simulink model "Filter_Fixed"  (R2017b)
settings: Solver=FixedStepDiscrete  StartTime=0.0  StopTime=400  RelTol=1e-3
undefined symbols (not defined in the file or in its folder): designMultirateFIR
libraries: dspmlti4 x1
(part 3 of 3)

== system Filter_Fixed/HighpassH/Resonator75 ==
  In1 : Inport
  Delay : Delay  DelayLength=1
  Gain : Gain  Gain=-0.9536+0.30107i  OutDataTypeStr=fixdt(1,24,23)
  GainH : Gain  Gain=-0.16604-0.98612i  OutDataTypeStr=fixdt(1,24,23)
  Sum1 : Sum  Inputs=|++
  Out1 : Outport
  wires:
  In1/1 -> Sum1/1
  GainH/1 -> Out1/1
  Gain/1 -> Sum1/2
  Delay/1 -> Gain/1
  Sum1/1 -> Delay/1, GainH/1

== system Filter_Fixed/HighpassH/Resonator76 ==
  In1 : Inport
  Delay : Delay  DelayLength=1
  Gain : Gain  Gain=-0.9616+0.27445i  OutDataTypeStr=fixdt(1,24,23)
  GainH : Gain  Gain=0.15231+0.98833i  OutDataTypeStr=fixdt(1,24,23)
  Sum1 : Sum  Inputs=|++
  Out1 : Outport
  wires:
  In1/1 -> Sum1/1
  GainH/1 -> Out1/1
  Gain/1 -> Sum1/2
  Delay/1 -> Gain/1
  Sum1/1 -> Delay/1, GainH/1

== system Filter_Fixed/HighpassH/Resonator77 ==
  In1 : Inport
  Delay : Delay  DelayLength=1
  Gain : Gain  Gain=-0.96886+0.24761i  OutDataTypeStr=fixdt(1,24,23)
  GainH : Gain  Gain=-0.13856-0.99035i  OutDataTypeStr=fixdt(1,24,23)
  Sum1 : Sum  Inputs=|++
  Out1 : Outport
  wires:
  In1/1 -> Sum1/1
  GainH/1 -> Out1/1
  Gain/1 -> Sum1/2
  Delay/1 -> Gain/1
  Sum1/1 -> Delay/1, GainH/1

== system Filter_Fixed/HighpassH/Resonator78 ==
  In1 : Inport
  Delay : Delay  DelayLength=1
  Gain : Gain  Gain=-0.97537+0.22058i  OutDataTypeStr=fixdt(1,24,23)
  GainH : Gain  Gain=0.12478+0.99218i  OutDataTypeStr=fixdt(1,24,23)
  Sum1 : Sum  Inputs=|++
  Out1 : Outport
  wires:
  In1/1 -> Sum1/1
  GainH/1 -> Out1/1
  Gain/1 -> Sum1/2
  Delay/1 -> Gain/1
  Sum1/1 -> Delay/1, GainH/1

== system Filter_Fixed/HighpassH/Resonator79 ==
  In1 : Inport
  Delay : Delay  DelayLength=1
  Gain : Gain  Gain=-0.98112+0.19339i  OutDataTypeStr=fixdt(1,24,23)
  GainH : Gain  Gain=-0.11098-0.99382i  OutDataTypeStr=fixdt(1,24,23)
  Sum1 : Sum  Inputs=|++
  Out1 : Outport
  wires:
  In1/1 -> Sum1/1
  GainH/1 -> Out1/1
  Gain/1 -> Sum1/2
  Delay/1 -> Gain/1
  Sum1/1 -> Delay/1, GainH/1

== system Filter_Fixed/HighpassH/Resonator8 ==
  In1 : Inport
  Delay : Delay  DelayLength=1
  Gain : Gain  Gain=0.56277+0.82661i  OutDataTypeStr=fixdt(1,24,23)
  GainH : Gain  Gain=0.89037+0.45523i  OutDataTypeStr=fixdt(1,24,23)
  Sum1 : Sum  Inputs=|++
  Out1 : Outport
  wires:
  In1/1 -> Sum1/1
  GainH/1 -> Out1/1
  Gain/1 -> Sum1/2
  Delay/1 -> Gain/1
  Sum1/1 -> Delay/1, GainH/1

== system Filter_Fixed/HighpassH/Resonator80 ==
  In1 : Inport
  Delay : Delay  DelayLength=1
  Gain : Gain  Gain=-0.98612+0.16604i  OutDataTypeStr=fixdt(1,24,23)
  GainH : Gain  Gain=0.097152+0.99527i  OutDataTypeStr=fixdt(1,24,23)
  Sum1 : Sum  Inputs=|++
  Out1 : Outport
  wires:
  In1/1 -> Sum1/1
  GainH/1 -> Out1/1
  Gain/1 -> Sum1/2
  Delay/1 -> Gain/1
  Sum1/1 -> Delay/1, GainH/1

== system Filter_Fixed/HighpassH/Resonator81 ==
  In1 : Inport
  Delay : Delay  DelayLength=1
  Gain : Gain  Gain=-0.99035+0.13856i  OutDataTypeStr=fixdt(1,24,23)
  GainH : Gain  Gain=-0.083308-0.99652i  OutDataTypeStr=fixdt(1,24,23)
  Sum1 : Sum  Inputs=|++
  Out1 : Outport
  wires:
  In1/1 -> Sum1/1
  GainH/1 -> Out1/1
  Gain/1 -> Sum1/2
  Delay/1 -> Gain/1
  Sum1/1 -> Delay/1, GainH/1

== system Filter_Fixed/HighpassH/Resonator82 ==
  In1 : Inport
  Delay : Delay  DelayLength=1
  Gain : Gain  Gain=-0.99382+0.11098i  OutDataTypeStr=fixdt(1,24,23)
  GainH : Gain  Gain=0.069448+0.99759i  OutDataTypeStr=fixdt(1,24,23)
  Sum1 : Sum  Inputs=|++
  Out1 : Outport
  wires:
  In1/1 -> Sum1/1
  GainH/1 -> Out1/1
  Gain/1 -> Sum1/2
  Delay/1 -> Gain/1
  Sum1/1 -> Delay/1, GainH/1

== system Filter_Fixed/HighpassH/Resonator83 ==
  In1 : Inport
  Delay : Delay  DelayLength=1
  Gain : Gain  Gain=-0.99652+0.083308i  OutDataTypeStr=fixdt(1,24,23)
  GainH : Gain  Gain=-0.055575-0.99845i  OutDataTypeStr=fixdt(1,24,23)
  Sum1 : Sum  Inputs=|++
  Out1 : Outport
  wires:
  In1/1 -> Sum1/1
  GainH/1 -> Out1/1
  Gain/1 -> Sum1/2
  Delay/1 -> Gain/1
  Sum1/1 -> Delay/1, GainH/1

== system Filter_Fixed/HighpassH/Resonator84 ==
  In1 : Inport
  Delay : Delay  DelayLength=1
  Gain : Gain  Gain=-0.99845+0.055575i  OutDataTypeStr=fixdt(1,24,23)
  GainH : Gain  Gain=0.04169+0.99913i  OutDataTypeStr=fixdt(1,24,23)
  Sum1 : Sum  Inputs=|++
  Out1 : Outport
  wires:
  In1/1 -> Sum1/1
  GainH/1 -> Out1/1
  Gain/1 -> Sum1/2
  Delay/1 -> Gain/1
  Sum1/1 -> Delay/1, GainH/1

== system Filter_Fixed/HighpassH/Resonator85 ==
  In1 : Inport
  Delay : Delay  DelayLength=1
  Gain : Gain  Gain=-0.99961+0.027798i  OutDataTypeStr=fixdt(1,24,23)
  GainH : Gain  Gain=-0.027798-0.99961i  OutDataTypeStr=fixdt(1,24,23)
  Sum1 : Sum  Inputs=|++
  Out1 : Outport
  wires:
  In1/1 -> Sum1/1
  GainH/1 -> Out1/1
  Gain/1 -> Sum1/2
  Delay/1 -> Gain/1
  Sum1/1 -> Delay/1, GainH/1

== system Filter_Fixed/HighpassH/Resonator86 ==
  In1 : Inport
  Delay : Delay  DelayLength=1
  Gain : Gain  Gain=-1+1.2246e-16i  OutDataTypeStr=fixdt(1,24,23)
  GainH : Gain  Gain=0.0139+0.9999i  OutDataTypeStr=fixdt(1,24,23)
  Sum1 : Sum  Inputs=|++
  Out1 : Outport
  wires:
  In1/1 -> Sum1/1
  GainH/1 -> Out1/1
  Gain/1 -> Sum1/2
  Delay/1 -> Gain/1
  Sum1/1 -> Delay/1, GainH/1

== system Filter_Fixed/HighpassH/Resonator87 ==
  In1 : Inport
  Delay : Delay  DelayLength=1
  Gain : Gain  Gain=-0.99961-0.027798i  OutDataTypeStr=fixdt(1,24,23)
  GainH : Gain  Gain=1.9106e-14-1i  OutDataTypeStr=fixdt(1,24,23)
  Sum1 : Sum  Inputs=|++
  Out1 : Outport
  wires:
  In1/1 -> Sum1/1
  GainH/1 -> Out1/1
  Gain/1 -> Sum1/2
  Delay/1 -> Gain/1
  Sum1/1 -> Delay/1, GainH/1

== system Filter_Fixed/HighpassH/Resonator88 ==
  In1 : Inport
  Delay : Delay  DelayLength=1
  Gain : Gain  Gain=-0.99845-0.055575i  OutDataTypeStr=fixdt(1,24,23)
  GainH : Gain  Gain=0.0139-0.9999i  OutDataTypeStr=fixdt(1,24,23)
  Sum1 : Sum  Inputs=|++
  Out1 : Outport
  wires:
  In1/1 -> Sum1/1
  GainH/1 -> Out1/1
  Gain/1 -> Sum1/2
  Delay/1 -> Gain/1
  Sum1/1 -> Delay/1, GainH/1

== system Filter_Fixed/HighpassH/Resonator89 ==
  In1 : Inport
  Delay : Delay  DelayLength=1
  Gain : Gain  Gain=-0.99652-0.083308i  OutDataTypeStr=fixdt(1,24,23)
  GainH : Gain  Gain=-0.027798+0.99961i  OutDataTypeStr=fixdt(1,24,23)
  Sum1 : Sum  Inputs=|++
  Out1 : Outport
  wires:
  In1/1 -> Sum1/1
  GainH/1 -> Out1/1
  Gain/1 -> Sum1/2
  Delay/1 -> Gain/1
  Sum1/1 -> Delay/1, GainH/1

== system Filter_Fixed/HighpassH/Resonator9 ==
  In1 : Inport
  Delay : Delay  DelayLength=1
  Gain : Gain  Gain=0.53958+0.84194i  OutDataTypeStr=fixdt(1,24,23)
  GainH : Gain  Gain=-0.88396-0.46756i  OutDataTypeStr=fixdt(1,24,23)
  Sum1 : Sum  Inputs=|++
  Out1 : Outport
  wires:
  In1/1 -> Sum1/1
  GainH/1 -> Out1/1
  Gain/1 -> Sum1/2
  Delay/1 -> Gain/1
  Sum1/1 -> Delay/1, GainH/1

== system Filter_Fixed/HighpassH/Resonator90 ==
  In1 : Inport
  Delay : Delay  DelayLength=1
  Gain : Gain  Gain=-0.99382-0.11098i  OutDataTypeStr=fixdt(1,24,23)
  GainH : Gain  Gain=0.04169-0.99913i  OutDataTypeStr=fixdt(1,24,23)
  Sum1 : Sum  Inputs=|++
  Out1 : Outport
  wires:
  In1/1 -> Sum1/1
  GainH/1 -> Out1/1
  Gain/1 -> Sum1/2
  Delay/1 -> Gain/1
  Sum1/1 -> Delay/1, GainH/1

== system Filter_Fixed/HighpassH/Resonator91 ==
  In1 : Inport
  Delay : Delay  DelayLength=1
  Gain : Gain  Gain=-0.99035-0.13856i  OutDataTypeStr=fixdt(1,24,23)
  GainH : Gain  Gain=-0.055575+0.99845i  OutDataTypeStr=fixdt(1,24,23)
  Sum1 : Sum  Inputs=|++
  Out1 : Outport
  wires:
  In1/1 -> Sum1/1
  GainH/1 -> Out1/1
  Gain/1 -> Sum1/2
  Delay/1 -> Gain/1
  Sum1/1 -> Delay/1, GainH/1

== system Filter_Fixed/HighpassH/Resonator92 ==
  In1 : Inport
  Delay : Delay  DelayLength=1
  Gain : Gain  Gain=-0.98612-0.16604i  OutDataTypeStr=fixdt(1,24,23)
  GainH : Gain  Gain=0.069448-0.99759i  OutDataTypeStr=fixdt(1,24,23)
  Sum1 : Sum  Inputs=|++
  Out1 : Outport
  wires:
  In1/1 -> Sum1/1
  GainH/1 -> Out1/1
  Gain/1 -> Sum1/2
  Delay/1 -> Gain/1
  Sum1/1 -> Delay/1, GainH/1

== system Filter_Fixed/HighpassH/Resonator93 ==
  In1 : Inport
  Delay : Delay  DelayLength=1
  Gain : Gain  Gain=-0.98112-0.19339i  OutDataTypeStr=fixdt(1,24,23)
  GainH : Gain  Gain=-0.083308+0.99652i  OutDataTypeStr=fixdt(1,24,23)
  Sum1 : Sum  Inputs=|++
  Out1 : Outport
  wires:
  In1/1 -> Sum1/1
  GainH/1 -> Out1/1
  Gain/1 -> Sum1/2
  Delay/1 -> Gain/1
  Sum1/1 -> Delay/1, GainH/1

== system Filter_Fixed/HighpassH/Resonator94 ==
  In1 : Inport
  Delay : Delay  DelayLength=1
  Gain : Gain  Gain=-0.97537-0.22058i  OutDataTypeStr=fixdt(1,24,23)
  GainH : Gain  Gain=0.097152-0.99527i  OutDataTypeStr=fixdt(1,24,23)
  Sum1 : Sum  Inputs=|++
  Out1 : Outport
  wires:
  In1/1 -> Sum1/1
  GainH/1 -> Out1/1
  Gain/1 -> Sum1/2
  Delay/1 -> Gain/1
  Sum1/1 -> Delay/1, GainH/1

== system Filter_Fixed/HighpassH/Resonator95 ==
  In1 : Inport
  Delay : Delay  DelayLength=1
  Gain : Gain  Gain=-0.96886-0.24761i  OutDataTypeStr=fixdt(1,24,23)
  GainH : Gain  Gain=-0.11098+0.99382i  OutDataTypeStr=fixdt(1,24,23)
  Sum1 : Sum  Inputs=|++
  Out1 : Outport
  wires:
  In1/1 -> Sum1/1
  GainH/1 -> Out1/1
  Gain/1 -> Sum1/2
  Delay/1 -> Gain/1
  Sum1/1 -> Delay/1, GainH/1

== system Filter_Fixed/HighpassH/Resonator96 ==
  In1 : Inport
  Delay : Delay  DelayLength=1
  Gain : Gain  Gain=-0.9616-0.27445i  OutDataTypeStr=fixdt(1,24,23)
  GainH : Gain  Gain=0.12478-0.99218i  OutDataTypeStr=fixdt(1,24,23)
  Sum1 : Sum  Inputs=|++
  Out1 : Outport
  wires:
  In1/1 -> Sum1/1
  GainH/1 -> Out1/1
  Gain/1 -> Sum1/2
  Delay/1 -> Gain/1
  Sum1/1 -> Delay/1, GainH/1

== system Filter_Fixed/HighpassH/Resonator97 ==
  In1 : Inport
  Delay : Delay  DelayLength=1
  Gain : Gain  Gain=-0.9536-0.30107i  OutDataTypeStr=fixdt(1,24,23)
  GainH : Gain  Gain=-0.13856+0.99035i  OutDataTypeStr=fixdt(1,24,23)
  Sum1 : Sum  Inputs=|++
  Out1 : Outport
  wires:
  In1/1 -> Sum1/1
  GainH/1 -> Out1/1
  Gain/1 -> Sum1/2
  Delay/1 -> Gain/1
  Sum1/1 -> Delay/1, GainH/1

== system Filter_Fixed/HighpassH/Resonator98 ==
  In1 : Inport
  Delay : Delay  DelayLength=1
  Gain : Gain  Gain=-0.94486-0.32747i  OutDataTypeStr=fixdt(1,24,23)
  GainH : Gain  Gain=0.15231-0.98833i  OutDataTypeStr=fixdt(1,24,23)
  Sum1 : Sum  Inputs=|++
  Out1 : Outport
  wires:
  In1/1 -> Sum1/1
  GainH/1 -> Out1/1
  Gain/1 -> Sum1/2
  Delay/1 -> Gain/1
  Sum1/1 -> Delay/1, GainH/1

== system Filter_Fixed/HighpassH/Resonator99 ==
  In1 : Inport
  Delay : Delay  DelayLength=1
  Gain : Gain  Gain=-0.93539-0.3536i  OutDataTypeStr=fixdt(1,24,23)
  GainH : Gain  Gain=-0.16604+0.98612i  OutDataTypeStr=fixdt(1,24,23)
  Sum1 : Sum  Inputs=|++
  Out1 : Outport
  wires:
  In1/1 -> Sum1/1
  GainH/1 -> Out1/1
  Gain/1 -> Sum1/2
  Delay/1 -> Gain/1
  Sum1/1 -> Delay/1, GainH/1

== system Filter_Fixed/HighpassH/ResonatorTemplate ==
  In1 : Inport
  Delay : Delay  DelayLength=1
  Gain : Gain
  GainH : Gain
  Sum1 : Sum  Inputs=|++
  Out1 : Outport
  wires:
  Sum1/1 -> GainH/1, Delay/1
  Delay/1 -> Gain/1
  Gain/1 -> Sum1/2
  GainH/1 -> Out1/1
  In1/1 -> Sum1/1

== system Filter_Fixed/LowpassH/Resonator1 ==
  In1 : Inport
  Delay : Delay  DelayLength=1
  Gain : Gain  Gain=0.99961+0.027798i  OutDataTypeStr=fixdt(1,24,23)
  GainH : Gain  OutDataTypeStr=fixdt(1,24,23)
  Sum1 : Sum  Inputs=|++
  Out1 : Outport
  wires:
  In1/1 -> Sum1/1
  GainH/1 -> Out1/1
  Gain/1 -> Sum1/2
  Delay/1 -> Gain/1
  Sum1/1 -> Delay/1, GainH/1

== system Filter_Fixed/LowpassH/Resonator10 ==
  In1 : Inport
  Delay : Delay  DelayLength=1
  Gain : Gain  Gain=0.9616+0.27445i  OutDataTypeStr=fixdt(1,24,23)
  GainH : Gain  Gain=0.72887-0.68465i  OutDataTypeStr=fixdt(1,24,23)
  Sum1 : Sum  Inputs=|++
  Out1 : Outport
  wires:
  In1/1 -> Sum1/1
  GainH/1 -> Out1/1
  Gain/1 -> Sum1/2
  Delay/1 -> Gain/1
  Sum1/1 -> Delay/1, GainH/1

== system Filter_Fixed/LowpassH/Resonator11 ==
  In1 : Inport
  Delay : Delay  DelayLength=1
  Gain : Gain  Gain=0.9536+0.30107i  OutDataTypeStr=fixdt(1,24,23)
  GainH : Gain  Gain=0.034745-0.9994i  OutDataTypeStr=fixdt(1,24,23)
  Sum1 : Sum  Inputs=|++
  Out1 : Outport
  wires:
  In1/1 -> Sum1/1
  GainH/1 -> Out1/1
  Gain/1 -> Sum1/2
  Delay/1 -> Gain/1
  Sum1/1 -> Delay/1, GainH/1

== system Filter_Fixed/LowpassH/Resonator12 ==
  In1 : Inport
  Delay : Delay  DelayLength=1
  Gain : Gain  Gain=0.94486+0.32747i  OutDataTypeStr=fixdt(1,24,23)
  GainH : Gain  Gain=-0.67957-0.73361i  OutDataTypeStr=fixdt(1,24,23)
  Sum1 : Sum  Inputs=|++
  Out1 : Outport
  wires:
  In1/1 -> Sum1/1
  GainH/1 -> Out1/1
  Gain/1 -> Sum1/2
  Delay/1 -> Gain/1
  Sum1/1 -> Delay/1, GainH/1

== system Filter_Fixed/LowpassH/Resonator13 ==
  In1 : Inport
  Delay : Delay  DelayLength=1
  Gain : Gain  Gain=0.9616-0.27445i  OutDataTypeStr=fixdt(1,24,23)
  GainH : Gain  Gain=-0.67957+0.73361i  OutDataTypeStr=fixdt(1,24,23)
  Sum1 : Sum  Inputs=|++
  Out1 : Outport
  wires:
  In1/1 -> Sum1/1
  GainH/1 -> Out1/1
  Gain/1 -> Sum1/2
  Delay/1 -> Gain/1
  Sum1/1 -> Delay/1, GainH/1

== system Filter_Fixed/LowpassH/Resonator14 ==
  In1 : Inport
  Delay : Delay  DelayLength=1
  Gain : Gain  Gain=0.96886-0.24761i  OutDataTypeStr=fixdt(1,24,23)
  GainH : Gain  Gain=0.034745+0.9994i  OutDataTypeStr=fixdt(1,24,23)
  Sum1 : Sum  Inputs=|++
  Out1 : Outport
  wires:
  In1/1 -> Sum1/1
  GainH/1 -> Out1/1
  Gain/1 -> Sum1/2
  Delay/1 -> Gain/1
  Sum1/1 -> Delay/1, GainH/1

== system Filter_Fixed/LowpassH/Resonator15 ==
  In1 : Inport
  Delay : Delay  DelayLength=1
  Gain : Gain  Gain=0.97537-0.22058i  OutDataTypeStr=fixdt(1,24,23)
  GainH : Gain  Gain=0.72887+0.68465i  OutDataTypeStr=fixdt(1,24,23)
  Sum1 : Sum  Inputs=|++
  Out1 : Outport
  wires:
  In1/1 -> Sum1/1
  GainH/1 -> Out1/1
  Gain/1 -> Sum1/2
  Delay/1 -> Gain/1
  Sum1/1 -> Delay/1, GainH/1

== system Filter_Fixed/LowpassH/Resonator16 ==
  In1 : Inport
  Delay : Delay  DelayLength=1
  Gain : Gain  Gain=0.98112-0.19339i  OutDataTypeStr=fixdt(1,24,23)
  GainH : Gain  Gain=0.99961-0.027798i  OutDataTypeStr=fixdt(1,24,23)
  Sum1 : Sum  Inputs=|++
  Out1 : Outport
  wires:
  In1/1 -> Sum1/1
  GainH/1 -> Out1/1
  Gain/1 -> Sum1/2
  Delay/1 -> Gain/1
  Sum1/1 -> Delay/1, GainH/1

== system Filter_Fixed/LowpassH/Resonator17 ==
  In1 : Inport
  Delay : Delay  DelayLength=1
  Gain : Gain  Gain=0.98612-0.16604i  OutDataTypeStr=fixdt(1,24,23)
  GainH : Gain  Gain=0.6897-0.7241i  OutDataTypeStr=fixdt(1,24,23)
  Sum1 : Sum  Inputs=|++
  Out1 : Outport
  wires:
  In1/1 -> Sum1/1
  GainH/1 -> Out1/1
  Gain/1 -> Sum1/2
  Delay/1 -> Gain/1
  Sum1/1 -> Delay/1, GainH/1

== system Filter_Fixed/LowpassH/Resonator18 ==
  In1 : Inport
  Delay : Delay  DelayLength=1
  Gain : Gain  Gain=0.99035-0.13856i  OutDataTypeStr=fixdt(1,24,23)
  GainH : Gain  Gain=-0.02085-0.99978i  OutDataTypeStr=fixdt(1,24,23)
  Sum1 : Sum  Inputs=|++
  Out1 : Outport
  wires:
  In1/1 -> Sum1/1
  GainH/1 -> Out1/1
  Gain/1 -> Sum1/2
  Delay/1 -> Gain/1
  Sum1/1 -> Delay/1, GainH/1

== system Filter_Fixed/LowpassH/Resonator19 ==
  In1 : Inport
  Delay : Delay  DelayLength=1
  Gain : Gain  Gain=0.99382-0.11098i  OutDataTypeStr=fixdt(1,24,23)
  GainH : Gain  Gain=-0.71929-0.69471i  OutDataTypeStr=fixdt(1,24,23)
  Sum1 : Sum  Inputs=|++
  Out1 : Outport
  wires:
  In1/1 -> Sum1/1
  GainH/1 -> Out1/1
  Gain/1 -> Sum1/2
  Delay/1 -> Gain/1
  Sum1/1 -> Delay/1, GainH/1

== system Filter_Fixed/LowpassH/Resonator2 ==
  In1 : Inport
  Delay : Delay  DelayLength=1
  Gain : Gain  Gain=0.99845+0.055575i  OutDataTypeStr=fixdt(1,24,23)
  GainH : Gain  Gain=0.70956-0.70465i  OutDataTypeStr=fixdt(1,24,23)
  Sum1 : Sum  Inputs=|++
  Out1 : Outport
  wires:
  In1/1 -> Sum1/1
  GainH/1 -> Out1/1
  Gain/1 -> Sum1/2
  Delay/1 -> Gain/1
  Sum1/1 -> Delay/1, GainH/1

== system Filter_Fixed/LowpassH/Resonator20 ==
  In1 : Inport
  Delay : Delay  DelayLength=1
  Gain : Gain  Gain=0.99652-0.083308i  OutDataTypeStr=fixdt(1,24,23)
  GainH : Gain  Gain=-0.9999+0.0139i  OutDataTypeStr=fixdt(1,24,23)
  Sum1 : Sum  Inputs=|++
  Out1 : Outport
  wires:
  In1/1 -> Sum1/1
  GainH/1 -> Out1/1
  Gain/1 -> Sum1/2
  Delay/1 -> Gain/1
  Sum1/1 -> Delay/1, GainH/1

== system Filter_Fixed/LowpassH/Resonator21 ==
  In1 : Inport
  Delay : Delay  DelayLength=1
  Gain : Gain  Gain=0.99845-0.055575i  OutDataTypeStr=fixdt(1,24,23)
  GainH : Gain  Gain=-0.6997+0.71444i  OutDataTypeStr=fixdt(1,24,23)
  Sum1 : Sum  Inputs=|++
  Out1 : Outport
  wires:
  In1/1 -> Sum1/1
  GainH/1 -> Out1/1
  Gain/1 -> Sum1/2
  Delay/1 -> Gain/1
  Sum1/1 -> Delay/1, GainH/1

== system Filter_Fixed/LowpassH/Resonator22 ==
  In1 : Inport
  Delay : Delay  DelayLength=1
  Gain : Gain  Gain=0.99961-0.027798i  OutDataTypeStr=fixdt(1,24,23)
  GainH : Gain  Gain=0.0069504+0.99998i  OutDataTypeStr=fixdt(1,24,23)
  Sum1 : Sum  Inputs=|++
  Out1 : Outport
  wires:
  In1/1 -> Sum1/1
  GainH/1 -> Out1/1
  Gain/1 -> Sum1/2
  Delay/1 -> Gain/1
  Sum1/1 -> Delay/1, GainH/1

== system Filter_Fixed/LowpassH/Resonator23 ==
  In1 : Inport
  Delay : Delay  DelayLength=1
  Gain : Gain  Gain=1-2.4493e-16i  OutDataTypeStr=fixdt(1,24,23)
  GainH : Gain  Gain=0.70956+0.70465i  OutDataTypeStr=fixdt(1,24,23)
  Sum1 : Sum  Inputs=|++
  Out1 : Outport
  wires:
  In1/1 -> Sum1/1
  GainH/1 -> Out1/1
  Gain/1 -> Sum1/2
  Delay/1 -> Gain/1
  Sum1/1 -> Delay/1, GainH/1

== system Filter_Fixed/LowpassH/Resonator3 ==
  In1 : Inport
  Delay : Delay  DelayLength=1
  Gain : Gain  Gain=0.99652+0.083308i  OutDataTypeStr=fixdt(1,24,23)
  GainH : Gain  Gain=0.0069504-0.99998i  OutDataTypeStr=fixdt(1,24,23)
  Sum1 : Sum  Inputs=|++
  Out1 : Outport
  wires:
  In1/1 -> Sum1/1
  GainH/1 -> Out1/1
  Gain/1 -> Sum1/2
  Delay/1 -> Gain/1
  Sum1/1 -> Delay/1, GainH/1

== system Filter_Fixed/LowpassH/Resonator4 ==
  In1 : Inport
  Delay : Delay  DelayLength=1
  Gain : Gain  Gain=0.99382+0.11098i  OutDataTypeStr=fixdt(1,24,23)
  GainH : Gain  Gain=-0.6997-0.71444i  OutDataTypeStr=fixdt(1,24,23)
  Sum1 : Sum  Inputs=|++
  Out1 : Outport
  wires:
  In1/1 -> Sum1/1
  GainH/1 -> Out1/1
  Gain/1 -> Sum1/2
  Delay/1 -> Gain/1
  Sum1/1 -> Delay/1, GainH/1

== system Filter_Fixed/LowpassH/Resonator5 ==
  In1 : Inport
  Delay : Delay  DelayLength=1
  Gain : Gain  Gain=0.99035+0.13856i  OutDataTypeStr=fixdt(1,24,23)
  GainH : Gain  Gain=-0.9999-0.0139i  OutDataTypeStr=fixdt(1,24,23)
  Sum1 : Sum  Inputs=|++
  Out1 : Outport
  wires:
  In1/1 -> Sum1/1
  GainH/1 -> Out1/1
  Gain/1 -> Sum1/2
  Delay/1 -> Gain/1
  Sum1/1 -> Delay/1, GainH/1

== system Filter_Fixed/LowpassH/Resonator6 ==
  In1 : Inport
  Delay : Delay  DelayLength=1
  Gain : Gain  Gain=0.98612+0.16604i  OutDataTypeStr=fixdt(1,24,23)
  GainH : Gain  Gain=-0.71929+0.69471i  OutDataTypeStr=fixdt(1,24,23)
  Sum1 : Sum  Inputs=|++
  Out1 : Outport
  wires:
  In1/1 -> Sum1/1
  GainH/1 -> Out1/1
  Gain/1 -> Sum1/2
  Delay/1 -> Gain/1
  Sum1/1 -> Delay/1, GainH/1

== system Filter_Fixed/LowpassH/Resonator7 ==
  In1 : Inport
  Delay : Delay  DelayLength=1
  Gain : Gain  Gain=0.98112+0.19339i  OutDataTypeStr=fixdt(1,24,23)
  GainH : Gain  Gain=-0.02085+0.99978i  OutDataTypeStr=fixdt(1,24,23)
  Sum1 : Sum  Inputs=|++
  Out1 : Outport
  wires:
  In1/1 -> Sum1/1
  GainH/1 -> Out1/1
  Gain/1 -> Sum1/2
  Delay/1 -> Gain/1
  Sum1/1 -> Delay/1, GainH/1

== system Filter_Fixed/LowpassH/Resonator8 ==
  In1 : Inport
  Delay : Delay  DelayLength=1
  Gain : Gain  Gain=0.97537+0.22058i  OutDataTypeStr=fixdt(1,24,23)
  GainH : Gain  Gain=0.6897+0.7241i  OutDataTypeStr=fixdt(1,24,23)
  Sum1 : Sum  Inputs=|++
  Out1 : Outport
  wires:
  In1/1 -> Sum1/1
  GainH/1 -> Out1/1
  Gain/1 -> Sum1/2
  Delay/1 -> Gain/1
  Sum1/1 -> Delay/1, GainH/1

== system Filter_Fixed/LowpassH/Resonator9 ==
  In1 : Inport
  Delay : Delay  DelayLength=1
  Gain : Gain  Gain=0.96886+0.24761i  OutDataTypeStr=fixdt(1,24,23)
  GainH : Gain  Gain=0.99961+0.027798i  OutDataTypeStr=fixdt(1,24,23)
  Sum1 : Sum  Inputs=|++
  Out1 : Outport
  wires:
  In1/1 -> Sum1/1
  GainH/1 -> Out1/1
  Gain/1 -> Sum1/2
  Delay/1 -> Gain/1
  Sum1/1 -> Delay/1, GainH/1

== system Filter_Fixed/LowpassH/ResonatorTemplate ==
  In1 : Inport
  Delay : Delay  DelayLength=1
  Gain : Gain
  GainH : Gain
  Sum1 : Sum  Inputs=|++
  Out1 : Outport
  wires:
  Sum1/1 -> GainH/1, Delay/1
  Delay/1 -> Gain/1
  Gain/1 -> Sum1/2
  GainH/1 -> Out1/1
  In1/1 -> Sum1/1
